simulink model "rl"  (R2024a)
settings: Solver=VariableStepAuto  StartTime=0.0  StopTime=10.0  RelTol=1e-3
settings Model: Creator=Admin  LastModifiedBy=Admin

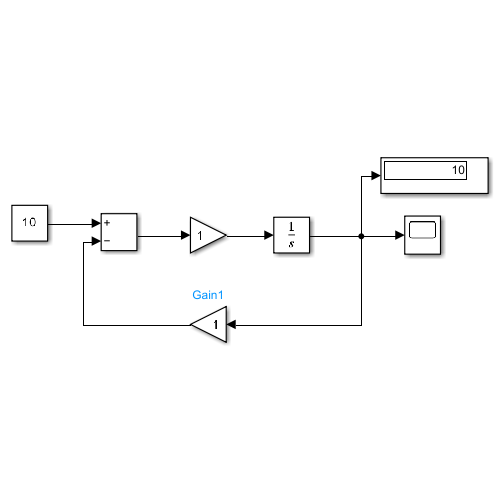
[thumbnail: Simulink's stored preview of the top-level diagram]
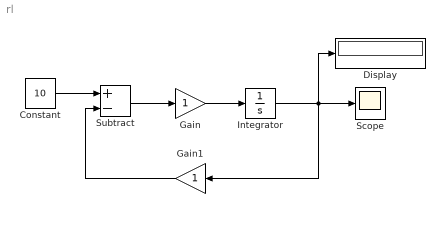
== system rl ==
  Constant : Constant  Value=10
  Display : Display
  Gain : Gain
  Gain1 : Gain
  Integrator : Integrator
  Scope : Scope
  Subtract : Sum  Inputs=+-
  wires:
  Gain/1 -> Integrator/1
  Subtract/1 -> Gain/1
  Constant/1 -> Subtract/1
  Integrator/1 -> Display/1, Scope/1, Gain1/1
  Gain1/1 -> Subtract/2
